simulink model "BEST2020_gamepad_template"  (R2019b)
settings: Solver=ode23t  StartTime=0.0  StopTime=180.1  FixedStep=0.05  RelTol=1e-3  EnableMultiTasking=on
model workspace (MAT data in the model file):
  mapForSim : object (value not decoded)
  occGrid : robotics.BinaryOccupancyGrid (value not decoded)
undefined symbols (not defined in the file): cellLevel, cellPose, cellTypeArray, FloorSurface, isoPoses, platformPoses, PlowSurface, Ref, RobotSurface, WallSurface, X, Y, Z
libraries: sm_lib x286, nesl_utility x158, simulink x72, vexcommonlib x1, vrlib x1
(part 14 of 14)

== matlab function BEST2020_gamepad_template/BEST Robotics 2020 Game (Double-Click)/Cells/Object18/MATLAB Function ==
  settings: updateMethod=DISCRETE
  data: latch input; scoreLevel input; inuse input; target input; time input; objPoseX output; robotPoseX input; robotPoseY input; objPoseY output; latched output; initPose parameter; objId parameter; cellType output; endType output; cellTypeArray parameter; gameTime parameter; platformPoses parameter; cellLevel parameter
function [objPoseX, objPoseY, latched, cellType,endType] = latchObject(latch,scoreLevel, inuse, target, time, robotPoseX, robotPoseY, initPose, objId, cellTypeArray, gameTime, platformPoses, cellLevel)
persistent stateX stateY level pickup
if isempty(stateX)
    stateX=initPose(1);
    stateY=initPose(2);
    level=cellLevel;
    pickup=0;
end

if ~latch
     pickup=0;
    if level && ((stateX > platformPoses(1,1)-0.21 && stateX < platformPoses(1,1)+0.21...
            && stateY > platformPoses(1,2)-0.21 && stateY < platformPoses(1,2) +0.21) || ...
            (stateX > platformPoses(2,1)-0.21 && stateX < platformPoses(2,1)+0.21...
            && stateY > platformPoses(2,2)-0.21 && stateY < platformPoses(2,2) +0.21))
        latched=0.4;
    else
        level=0;
        latched=0;
    end
elseif pickup
    stateX=robotPoseX;
    stateY=robotPoseY;
    level=scoreLevel;
    latched=0.15 +level*0.4;
elseif ~inuse && latch && target == objId && ...
        sqrt((stateX-robotPoseX)^2+(stateY-robotPoseY)^2) < 0.08 && scoreLevel==level
    
        pickup=1;
        latched=0.15;
else
   if level && ((stateX > platformPoses(1,1)-0.21 && stateX < platformPoses(1,1)+0.21...
            && stateY > platformPoses(1,2)-0.21 && stateY < platformPoses(1,2) +0.21) || ...
            (stateX > platformPoses(2,1)-0.21 && stateX < platformPoses(2,1)+0.21...
            && stateY > platformPoses(2,2)-0.21 && stateY < platformPoses(2,2) +0.21))
        latched=0.4;
    else
        level=0;
        latched=0;
    end
end
if sqrt((stateX-robotPoseX)^2+(stateY-robotPoseY)^2) < 0.1 && scoreLevel==level
    cellType=cellTypeArray(objId);
else
    cellType=nan;
end

if time > gameTime
    endType=cellTypeArray(objId)+1;
else
    endType=0;
end

objPoseX=stateX;
objPoseY=stateY;

== matlab function BEST2020_gamepad_template/BEST Robotics 2020 Game (Double-Click)/Cells/Object19/MATLAB Function ==
  settings: updateMethod=DISCRETE
  data: latch input; scoreLevel input; inuse input; target input; time input; objPoseX output; robotPoseX input; robotPoseY input; objPoseY output; latched output; initPose parameter; objId parameter; cellType output; endType output; cellTypeArray parameter; gameTime parameter; platformPoses parameter; cellLevel parameter
function [objPoseX, objPoseY, latched, cellType,endType] = latchObject(latch,scoreLevel, inuse, target, time, robotPoseX, robotPoseY, initPose, objId, cellTypeArray, gameTime, platformPoses, cellLevel)
persistent stateX stateY level pickup
if isempty(stateX)
    stateX=initPose(1);
    stateY=initPose(2);
    level=cellLevel;
    pickup=0;
end

if ~latch
     pickup=0;
    if level && ((stateX > platformPoses(1,1)-0.21 && stateX < platformPoses(1,1)+0.21...
            && stateY > platformPoses(1,2)-0.21 && stateY < platformPoses(1,2) +0.21) || ...
            (stateX > platformPoses(2,1)-0.21 && stateX < platformPoses(2,1)+0.21...
            && stateY > platformPoses(2,2)-0.21 && stateY < platformPoses(2,2) +0.21))
        latched=0.4;
    else
        level=0;
        latched=0;
    end
elseif pickup
    stateX=robotPoseX;
    stateY=robotPoseY;
    level=scoreLevel;
    latched=0.15 +level*0.4;
elseif ~inuse && latch && target == objId && ...
        sqrt((stateX-robotPoseX)^2+(stateY-robotPoseY)^2) < 0.08 && scoreLevel==level
    
        pickup=1;
        latched=0.15;
else
   if level && ((stateX > platformPoses(1,1)-0.21 && stateX < platformPoses(1,1)+0.21...
            && stateY > platformPoses(1,2)-0.21 && stateY < platformPoses(1,2) +0.21) || ...
            (stateX > platformPoses(2,1)-0.21 && stateX < platformPoses(2,1)+0.21...
            && stateY > platformPoses(2,2)-0.21 && stateY < platformPoses(2,2) +0.21))
        latched=0.4;
    else
        level=0;
        latched=0;
    end
end
if sqrt((stateX-robotPoseX)^2+(stateY-robotPoseY)^2) < 0.1 && scoreLevel==level
    cellType=cellTypeArray(objId);
else
    cellType=nan;
end

if time > gameTime
    endType=cellTypeArray(objId)+1;
else
    endType=0;
end

objPoseX=stateX;
objPoseY=stateY;

== matlab function BEST2020_gamepad_template/BEST Robotics 2020 Game (Double-Click)/Cells/Object20/MATLAB Function ==
  settings: updateMethod=DISCRETE
  data: latch input; scoreLevel input; inuse input; target input; time input; objPoseX output; robotPoseX input; robotPoseY input; objPoseY output; latched output; initPose parameter; objId parameter; cellType output; endType output; cellTypeArray parameter; gameTime parameter; platformPoses parameter; cellLevel parameter
function [objPoseX, objPoseY, latched, cellType,endType] = latchObject(latch,scoreLevel, inuse, target, time, robotPoseX, robotPoseY, initPose, objId, cellTypeArray, gameTime, platformPoses, cellLevel)
persistent stateX stateY level pickup
if isempty(stateX)
    stateX=initPose(1);
    stateY=initPose(2);
    level=cellLevel;
    pickup=0;
end

if ~latch
     pickup=0;
    if level && ((stateX > platformPoses(1,1)-0.21 && stateX < platformPoses(1,1)+0.21...
            && stateY > platformPoses(1,2)-0.21 && stateY < platformPoses(1,2) +0.21) || ...
            (stateX > platformPoses(2,1)-0.21 && stateX < platformPoses(2,1)+0.21...
            && stateY > platformPoses(2,2)-0.21 && stateY < platformPoses(2,2) +0.21))
        latched=0.4;
    else
        level=0;
        latched=0;
    end
elseif pickup
    stateX=robotPoseX;
    stateY=robotPoseY;
    level=scoreLevel;
    latched=0.15 +level*0.4;
elseif ~inuse && latch && target == objId && ...
        sqrt((stateX-robotPoseX)^2+(stateY-robotPoseY)^2) < 0.08 && scoreLevel==level
    
        pickup=1;
        latched=0.15;
else
   if level && ((stateX > platformPoses(1,1)-0.21 && stateX < platformPoses(1,1)+0.21...
            && stateY > platformPoses(1,2)-0.21 && stateY < platformPoses(1,2) +0.21) || ...
            (stateX > platformPoses(2,1)-0.21 && stateX < platformPoses(2,1)+0.21...
            && stateY > platformPoses(2,2)-0.21 && stateY < platformPoses(2,2) +0.21))
        latched=0.4;
    else
        level=0;
        latched=0;
    end
end
if sqrt((stateX-robotPoseX)^2+(stateY-robotPoseY)^2) < 0.1 && scoreLevel==level
    cellType=cellTypeArray(objId);
else
    cellType=nan;
end

if time > gameTime
    endType=cellTypeArray(objId)+1;
else
    endType=0;
end

objPoseX=stateX;
objPoseY=stateY;

== matlab function BEST2020_gamepad_template/BEST Robotics 2020 Game (Double-Click)/Cells/Object21/MATLAB Function ==
  settings: updateMethod=DISCRETE
  data: latch input; scoreLevel input; inuse input; target input; time input; objPoseX output; robotPoseX input; robotPoseY input; objPoseY output; latched output; initPose parameter; objId parameter; cellType output; endType output; cellTypeArray parameter; gameTime parameter; platformPoses parameter; cellLevel parameter
function [objPoseX, objPoseY, latched, cellType,endType] = latchObject(latch,scoreLevel, inuse, target, time, robotPoseX, robotPoseY, initPose, objId, cellTypeArray, gameTime, platformPoses, cellLevel)
persistent stateX stateY level pickup
if isempty(stateX)
    stateX=initPose(1);
    stateY=initPose(2);
    level=cellLevel;
    pickup=0;
end

if ~latch
     pickup=0;
    if level && ((stateX > platformPoses(1,1)-0.21 && stateX < platformPoses(1,1)+0.21...
            && stateY > platformPoses(1,2)-0.21 && stateY < platformPoses(1,2) +0.21) || ...
            (stateX > platformPoses(2,1)-0.21 && stateX < platformPoses(2,1)+0.21...
            && stateY > platformPoses(2,2)-0.21 && stateY < platformPoses(2,2) +0.21))
        latched=0.4;
    else
        level=0;
        latched=0;
    end
elseif pickup
    stateX=robotPoseX;
    stateY=robotPoseY;
    level=scoreLevel;
    latched=0.15 +level*0.4;
elseif ~inuse && latch && target == objId && ...
        sqrt((stateX-robotPoseX)^2+(stateY-robotPoseY)^2) < 0.08 && scoreLevel==level
    
        pickup=1;
        latched=0.15;
else
   if level && ((stateX > platformPoses(1,1)-0.21 && stateX < platformPoses(1,1)+0.21...
            && stateY > platformPoses(1,2)-0.21 && stateY < platformPoses(1,2) +0.21) || ...
            (stateX > platformPoses(2,1)-0.21 && stateX < platformPoses(2,1)+0.21...
            && stateY > platformPoses(2,2)-0.21 && stateY < platformPoses(2,2) +0.21))
        latched=0.4;
    else
        level=0;
        latched=0;
    end
end
if sqrt((stateX-robotPoseX)^2+(stateY-robotPoseY)^2) < 0.1 && scoreLevel==level
    cellType=cellTypeArray(objId);
else
    cellType=nan;
end

if time > gameTime
    endType=cellTypeArray(objId)+1;
else
    endType=0;
end

objPoseX=stateX;
objPoseY=stateY;

== matlab function BEST2020_gamepad_template/BEST Robotics 2020 Game (Double-Click)/Cells/MATLAB Function2 ==
  data: robotPose input; cellPoses input; cellTarget output
function cellTarget = findTarget(robotPose, cellPoses)


eucDist=sqrt((cellPoses(:,1)-robotPose(1)).^2+(cellPoses(:,2)-robotPose(2)).^2);
[~,cellIdx]=min(eucDist);
cellTarget = cellIdx;

== matlab function BEST2020_gamepad_template/BEST Robotics 2020 Game (Double-Click)/Vaccines/Vaccine/MATLAB Function ==
  settings: updateMethod=DISCRETE
  data: drop input; level input; objPoseX output; robotPoseX input; robotPoseY input; objPoseY output; vaccine output
function [objPoseX, objPoseY, vaccine] = latchObject(drop, level, robotPoseX, robotPoseY)
persistent stateX stateY stateZ prevDrop dropped
if isempty(stateX)
    stateX=robotPoseX+0.14;
    stateY=robotPoseY;
    stateZ=0.15;
    prevDrop=0;
    dropped=0;
end

if drop && prevDrop && ~dropped
    stateX=robotPoseX;
    stateY=robotPoseY;
    stateZ=level*0.4;
    objPoseX=robotPoseX;
    objPoseY=robotPoseY;
    dropped=1;
elseif dropped
    objPoseX=stateX;
    objPoseY=stateY;

else
    objPoseX=robotPoseX+0.14;
    objPoseY=robotPoseY;
end
prevDrop=drop;
vaccine=stateZ;

== matlab function BEST2020_gamepad_template/BEST Robotics 2020 Game (Double-Click)/Vaccines/Vaccine2/MATLAB Function1 ==
  settings: updateMethod=DISCRETE
  data: drop input; level input; objPoseX output; robotPoseX input; robotPoseY input; objPoseY output; vaccine output
function [objPoseX, objPoseY, vaccine] = latchObject(drop, level, robotPoseX, robotPoseY)
persistent stateX stateY stateZ prevDrop dropped
if isempty(stateX)
    stateX=robotPoseX+0.14;
    stateY=robotPoseY;
    stateZ=0.15;
    prevDrop=0;
    dropped=0;
end

if drop && prevDrop && ~dropped
    stateX=robotPoseX;
    stateY=robotPoseY;
    stateZ=level*0.4;
    objPoseX=robotPoseX;
    objPoseY=robotPoseY;
    dropped=1;
elseif dropped
    objPoseX=stateX;
    objPoseY=stateY;

else
    objPoseX=robotPoseX-0.11;
    objPoseY=robotPoseY+0.11;
end
prevDrop=drop;
vaccine=stateZ;

== matlab function BEST2020_gamepad_template/BEST Robotics 2020 Game (Double-Click)/Vaccines/Vaccine1/MATLAB Function1 ==
  settings: updateMethod=DISCRETE
  data: drop input; level input; objPoseX output; robotPoseX input; robotPoseY input; objPoseY output; vaccine output
function [objPoseX, objPoseY, vaccine] = latchObject(drop, level, robotPoseX, robotPoseY)
persistent stateX stateY stateZ prevDrop dropped
if isempty(stateX)
    stateX=robotPoseX+0.14;
    stateY=robotPoseY;
    stateZ=0.15;
    prevDrop=0;
    dropped=0;
end

if drop && prevDrop && ~dropped
    stateX=robotPoseX;
    stateY=robotPoseY;
    stateZ=level*0.4;
    objPoseX=robotPoseX;
    objPoseY=robotPoseY;
    dropped=1;
elseif dropped
    objPoseX=stateX;
    objPoseY=stateY;

else
    objPoseX=robotPoseX-0.11;
    objPoseY=robotPoseY-0.11;
end
prevDrop=drop;
vaccine=stateZ;
